simulink model "gm_slrt_pmsm_npc_inverter_slrt"  (R2022b)
settings: Solver=FixedStepAuto  StartTime=0.0  StopTime=0.25  RelTol=1e-3  EnableMultiTasking=on
PreLoadFcn:
  | Tcpu = 50e-6; %Controller sample time
  | 
  | % PMSM parameters
  | PM = 0.03; % Permanent magnet flux linkage
  | Ld = 2e-4;  % d-axis inductance
  | Lq = 2e-4;  % q-axis inductance
  | L0 = 2e-4;  % 0-axis inductance
  | Rs = 0.013; % Stator resistance
  | N = 6; % Number of pole pairs
  | J = 0.2; % Moment of inertia
  | 
  | % encoder parameters
  | numSlits = 2000; % number of slits
  | pulseSigOffset = 0; % index pulse signal offset
  | shaftInitPos = 0; % motor shaft initial position
  | 
  | % DAC parameters
  | gain = 0.1;
  | bias = 0;
  | 
  | % circuit parameters
  | Vdc = 48;
  | 
  | % Real-time processor or embedded controller
  | RTorTTL = 1; % 1: Real-time processor,    0: embedded controller
  | 
  | % real-time parameters
  | f_base = 200e6;
  | PWM_frequency = 20e3;
  | ts_FPGA_clk = 1/f_base;%5e-9
  | ts_FPGA_mdl =1e-6;
undefined symbols (not defined in the file or in its folder): IO334
libraries: speedgoatlib_hdlCoder_IO3xx x28, slrtencoderlib x1, slrtresolverlib x1
settings Model: Creator=chrisz  LastModifiedBy=chrisz
settings SolverCC: ConcurrentTasks=on  PositivePriorityOrder=on
settings OptimizationCC: BlockReduction=off  ConditionallyExecuteInputs=off  DefaultParameterBehavior=Inlined  OptimizeBlockIOStorage=off
settings DebuggingCC: AlgebraicLoopMsg=error  SingleTaskRateTransMsg=error  TasksWithSamePriorityMsg=none
settings HardwareCC: ProdBitPerLong=64  ProdLongLongMode=on  ProdHWDeviceType=Intel->x86-64 (Linux 64)  TargetBitPerPointer=64  TargetBitPerSizeT=64  TargetBitPerPtrDiffT=64  TargetLongLongMode=on  TargetIntDivRoundTo=Zero  TargetEndianess=LittleEndian  TargetWordSize=64  TargetHWDeviceType=Custom Processor->MATLAB Host Computer
settings ModelReferenceCC: EnableRefExpFcnMdlSchedulingChecks=on
settings RTWCC: Description=Simulink Real-Time  SystemTargetFile=slrealtime.tlc  TemplateMakefile=slrealtime_default_tmf  Toolchain=Simulink Real-Time Toolchain  BuildConfiguration=Faster Runs  CodeExecutionProfiling=on  TargetLang=C++

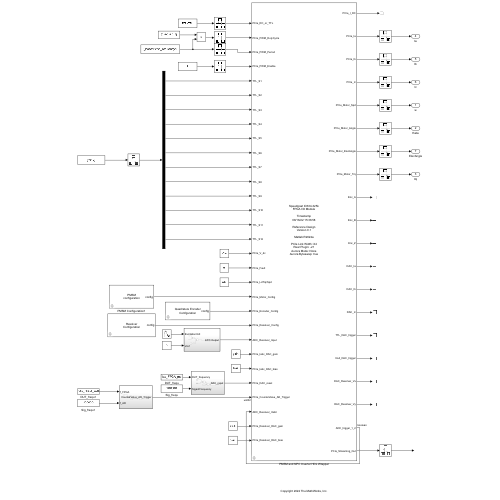
[thumbnail: Simulink's stored preview of the top-level diagram]
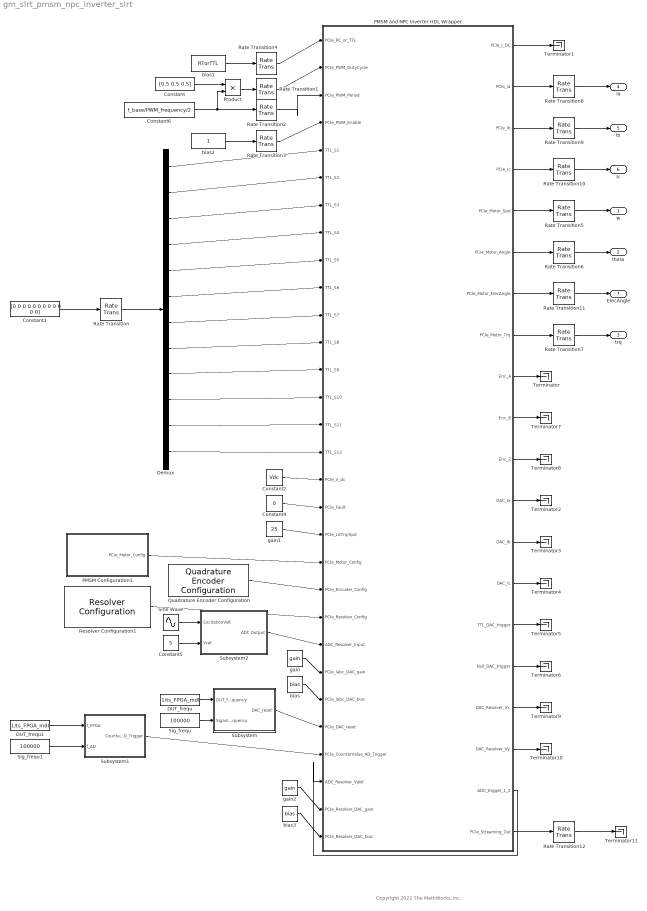
== system gm_slrt_pmsm_npc_inverter_slrt ==
  note: Copyright 2022 The MathWorks, Inc.
  Constant : Constant  Value=[0.5 0.5 0.5]  OutDataTypeStr=single  SampleTime=Tcpu
  Constant1 : Constant  Value=[0 0 0 0 0 0 0 0 0 0 0 0]  OutDataTypeStr=boolean  SampleTime=-1
  Constant2 : Constant  Value=Vdc  OutDataTypeStr=single  SampleTime=Tcpu
  Constant4 : Constant  Value=0  OutDataTypeStr=uint32  SampleTime=Tcpu
  Constant5 : Constant  Value=5  SampleTime=Tcpu
  Constant6 : Constant  Value=f_base/PWM_frequency/2  OutDataTypeStr=uint32  SampleTime=Tcpu
  DUT_frequ : Constant  Value=1/ts_FPGA_mdl  SampleTime=Tcpu
  DUT_frequ1 : Constant  Value=1/ts_FPGA_mdl  SampleTime=Tcpu
  Demux : Demux  Outputs=12
  PMSM Configuration1 : Subsystem  mask(PMSMConfig){portConfig=Torque, Trq_N_mode=0, Ts=Tcpu, Pp=4, Rs=0.02, Ld=1.7e-3, Lq=3.2e-3, lambda_pm=0.2205, J=0.0027, B=4.924e-4, f=0}
      mask prompts: portConfig "Mechanical input configuration:"; Ts "Sample time (s):"; Pp "Number of pole pairs:"; Rs "Stator resistance per phase (Ohm):"; Ld "Stator d-axis inductance (H):"; Lq "Stator q-axis inductance (H):"; lambda_pm "Permanent magnet flux linkage (Wb):"; J "Inertia (kgm^2):"; B "Viscous damping (Nm/rad/s):"; f "Static friction (Nm):"
      mask help: PMSM system configuration block
      mask TypeOptions portConfig: Torque | Speed
      mask Callback portConfig:
      | % Check the value selected in the pop-up
      | mask = Simulink.Mask.get(gcb);
      | portConfigStr = get_param(gcb, 'portConfig');
      | if strcmp(portConfigStr, 'Torque')
      |     % Set Trq_N_mode value to 0
      |     mask.getParameter('Trq_N_mode').Value = '0';
      | 
      | elseif strcmp(portConfigStr, 'Speed')
      |     % Set Trq_N_mode value to 2
      |     mask.getParameter('Trq_N_mode').Value = '1';
      | 
      | end
      mask DialogControl ParameterGroupVar Prompt: Block options
      mask DialogControl Container4 Prompt: Parameters
      mask Display:
      | disp('PMSM\nconfiguration');
      | port_label('output',1,'config');
  PMSM and NPC Inverter HDL Wrapper : Subsystem  mask(Speedgoat IO334-325k Interface Block){module_id=1, slot=-1, ts=-1, OutputRange=Auto (same as ADC), PullRPort0=pull-down, VioPort0=3.3V, PullRPort1=pull-down, VioPort1=3.3V, PullRPort2=pull-down, VioPort2=3.3V, PullRPort3=pull-down, VioPort3=3.3V, PullRPort4=pull-down, VioPort4=3.3V, PullRPort5=pull-down, VioPort5=3.3V, PullRPort6=pull-down, VioPort6=3.3V, FpgaFreq=200}
      mask prompts: module_id "FPGA Module Identifier:"; slot "PCI slot (-1: autosearch):"; ts "Sample time:"; OutputRange "DAC Voltage Range:"; PullRPort0 "pull resistor"; VioPort0 "I/O voltage"; PullRPort1 "pull resistor"; VioPort1 "I/O voltage"; PullRPort2 "pull resistor"; VioPort2 "I/O voltage"; PullRPort3 "pull resistor"; VioPort3 "I/O voltage"; PullRPort4 "pull resistor"; VioPort4 "I/O voltage"; PullRPort5 "pull resistor"; VioPort5 "I/O voltage"; PullRPort6 "pull resistor"; VioPort6 "I/O voltage"; FpgaFreq "FPGA Frequency [MHz]"
      mask help: Simulink Real-Time Interface Block for Speedgoat IO334-325k.
      mask init:
      | hdlslrt.backend.mfpgaparameters;
      mask Help: eval('speedgoatdoc_hdlc')
      mask TypeOptions OutputRange: IO334 DAC Setup/OutputRange
      mask TypeOptions PullRPort0: Port Settings -2x/PullRPort0
      mask Callback PullRPort0: sg_fpga_HDLCoder_io3xx_2x_m(2)
      mask TypeOptions VioPort0: Port Settings -2x/VioPort0
      mask Callback VioPort0: sg_fpga_HDLCoder_io3xx_2x_m(2)
      mask TypeOptions PullRPort1: Port Settings -2x/PullRPort1
      mask Callback PullRPort1: sg_fpga_HDLCoder_io3xx_2x_m(2)
      mask TypeOptions VioPort1: Port Settings -2x/VioPort1
      mask Callback VioPort1: sg_fpga_HDLCoder_io3xx_2x_m(2)
      mask TypeOptions PullRPort2: Port Settings -2x/PullRPort2
      mask Callback PullRPort2: sg_fpga_HDLCoder_io3xx_2x_m(2)
      mask TypeOptions VioPort2: Port Settings -2x/VioPort2
      mask Callback VioPort2: sg_fpga_HDLCoder_io3xx_2x_m(2)
      mask TypeOptions PullRPort3: Port Settings -2x/PullRPort3
      mask Callback PullRPort3: sg_fpga_HDLCoder_io3xx_2x_m(2)
      mask TypeOptions VioPort3: Port Settings -2x/VioPort3
      mask Callback VioPort3: sg_fpga_HDLCoder_io3xx_2x_m(2)
      mask TypeOptions PullRPort4: Port Settings -2x/PullRPort4
      mask Callback PullRPort4: sg_fpga_HDLCoder_io3xx_2x_m(2)
      mask TypeOptions VioPort4: Port Settings -2x/VioPort4
      mask Callback VioPort4: sg_fpga_HDLCoder_io3xx_2x_m(2)
      mask TypeOptions PullRPort5: Port Settings -2x/PullRPort5
      mask Callback PullRPort5: sg_fpga_HDLCoder_io3xx_2x_m(2)
      mask TypeOptions VioPort5: Port Settings -2x/VioPort5
      mask Callback VioPort5: sg_fpga_HDLCoder_io3xx_2x_m(2)
      mask TypeOptions PullRPort6: Port Settings -2x/PullRPort6
      mask Callback PullRPort6: sg_fpga_HDLCoder_io3xx_2x_m(2)
      mask TypeOptions VioPort6: Port Settings -2x/VioPort6
      mask Callback VioPort6: sg_fpga_HDLCoder_io3xx_2x_m(2)
      mask DialogControl AnalogOutput Prompt: Analog Output
      mask DialogControl IO33421 Prompt: IO334-21
      mask DialogControl port1 Prompt: Port 1
      mask DialogControl port2 Prompt: Port 2
      mask DialogControl port3 Prompt: Port 3
      mask DialogControl port4 Prompt: Port 4
      mask DialogControl port5 Prompt: Port 5
      mask DialogControl port6 Prompt: Port 6
      mask DialogControl port7 Prompt: Port 7
      mask Display:
      | SetupBlkPath = find_system(gcb, 'LookUnderMasks', 'all', 'FollowLinks', 'on', 'regexp', 'on', 'Name', 'IO3(\d|x){2}\s+Setup' );
      | SetupBlkPath = SetupBlkPath{1};
      | TS = get_param(SetupBlkPath,'timestamp_mcs');
      | disp(sprintf('Speedgoat IO334-325k\nFPGA I/O Module\n\nTimestamp\n%s\n\nReference Design\nVersion 0.1\n\nMatlab R2022a\n\nPCIe Link Width: X4\nRear Plugin: -21\nAurora Mode: None\nAurora Byteswap: true\n', TS))
  Product : Product  OutDataTypeStr=uint32
  Quadrature Encoder Configuration : slrtencoderlib/Quadrature Encoder Configuration  NPulses=2000  zOffset=0  Ts=Tcpu
  Rate Transition{,1..12} (13 alike) : RateTransition  OutPortSampleTime=Tcpu
  Resolver Configuration1 : slrtresolverlib/Resolver Configuration  Ts=Tcpu  R=0.5  N=1  ADCrefV=5  ADCbits=12  totalADCCounts=4096
  Sig_frequ : Constant  Value=100000  VectorParams1D=off  SampleTime=Tcpu
  Sig_frequ1 : Constant  Value=100000  VectorParams1D=off  SampleTime=Tcpu
  Sine Wave : Sin  Amplitude=5  Frequency=62830  SampleTime=Tcpu
  Subsystem : Subsystem
  Subsystem1 : Subsystem
  Subsystem2 : Subsystem
  Terminator{,1..11} (12 alike) : Terminator
  bias : Constant  Value=bias  OutDataTypeStr=single  SampleTime=Tcpu
  bias1 : Constant  Value=RTorTTL  OutDataTypeStr=single  SampleTime=Tcpu
  bias2 : Constant  OutDataTypeStr=boolean  SampleTime=Tcpu
  bias3 : Constant  Value=bias  OutDataTypeStr=single  SampleTime=Tcpu
  gain : Constant  Value=gain  OutDataTypeStr=single  SampleTime=Tcpu
  gain1 : Constant  Value=25  OutDataTypeStr=single  SampleTime=Tcpu
  gain2 : Constant  Value=gain  OutDataTypeStr=single  SampleTime=Tcpu
  w : Outport
  theta : Outport  Port=2
  trq : Outport  Port=3
  Ia : Outport  Port=4
  Ib : Outport  Port=5
  Ic : Outport  Port=6
  ElecAngle : Outport  Port=7
  wires:
  Rate Transition12/1 -> Terminator11/1
  PMSM and NPC Inverter HDL Wrapper/20(PCIe_Streaming_Out) -> Rate Transition12/1
  Rate Transition4/1 -> PMSM and NPC Inverter HDL Wrapper/1(PCIe_RC_or_TTL)
  Rate Transition1/1 -> PMSM and NPC Inverter HDL Wrapper/2(PCIe_PWM_DutyCycle)
  Rate Transition2/1 -> PMSM and NPC Inverter HDL Wrapper/3(PCIe_PWM_Period)
  Rate Transition3/1 -> PMSM and NPC Inverter HDL Wrapper/4(PCIe_PWM_Enable)
  Product/1 -> Rate Transition1/1
  Constant/1 -> Product/1
  bias2/1 -> Rate Transition3/1
  bias1/1 -> Rate Transition4/1
  Constant6/1 -> Rate Transition2/1, Product/2
  Demux/12 -> PMSM and NPC Inverter HDL Wrapper/16(TTL_S12)
  Demux/11 -> PMSM and NPC Inverter HDL Wrapper/15(TTL_S11)
  Demux/10 -> PMSM and NPC Inverter HDL Wrapper/14(TTL_S10)
  Demux/9 -> PMSM and NPC Inverter HDL Wrapper/13(TTL_S9)
  Demux/8 -> PMSM and NPC Inverter HDL Wrapper/12(TTL_S8)
  Demux/7 -> PMSM and NPC Inverter HDL Wrapper/11(TTL_S7)
  bias3/1 -> PMSM and NPC Inverter HDL Wrapper/30(PCIe_Resolver_DAC_bias)
  gain2/1 -> PMSM and NPC Inverter HDL Wrapper/29(PCIe_Resolver_DAC_gain)
  PMSM and NPC Inverter HDL Wrapper/7(PCIe_Motor_ElecAngle) -> Rate Transition11/1
  Rate Transition11/1 -> ElecAngle/1
  Subsystem2/1(ADC Output) -> PMSM and NPC Inverter HDL Wrapper/23(ADC_Resolver_Input)
  Constant5/1 -> Subsystem2/2(Vref)
  Sine Wave/1 -> Subsystem2/1(ExcitationVolt)
  DUT_frequ1/1 -> Subsystem1/1(f_FPGA)
  Sig_frequ1/1 -> Subsystem1/2(f_AD)
  PMSM and NPC Inverter HDL Wrapper/19(ADC_trigger_1_2) -> PMSM and NPC Inverter HDL Wrapper/28(ADC_Resolver_Valid)
  Subsystem1/1(CounterValue_AD_Trigger) -> PMSM and NPC Inverter HDL Wrapper/27(PCIe_CounterValue_AD_Trigger)
  Resolver Configuration1/1 -> PMSM and NPC Inverter HDL Wrapper/22(PCIe_Resolver_Config)
  PMSM Configuration1/1(PCIe_Motor_Config) -> PMSM and NPC Inverter HDL Wrapper/20(PCIe_Motor_Config)
  Quadrature Encoder Configuration/1 -> PMSM and NPC Inverter HDL Wrapper/21(PCIe_Encoder_Config)
  PMSM and NPC Inverter HDL Wrapper/18(DAC_Resolver_Vy) -> Terminator10/1
  PMSM and NPC Inverter HDL Wrapper/17(DAC_Resolver_Vx) -> Terminator9/1
  PMSM and NPC Inverter HDL Wrapper/11(Enc_Z) -> Terminator8/1
  PMSM and NPC Inverter HDL Wrapper/4(PCIe_Ic) -> Rate Transition10/1
  PMSM and NPC Inverter HDL Wrapper/3(PCIe_Ib) -> Rate Transition9/1
  PMSM and NPC Inverter HDL Wrapper/2(PCIe_Ia) -> Rate Transition8/1
  PMSM and NPC Inverter HDL Wrapper/8(PCIe_Motor_Trq) -> Rate Transition7/1
  PMSM and NPC Inverter HDL Wrapper/6(PCIe_Motor_Angle) -> Rate Transition6/1
  PMSM and NPC Inverter HDL Wrapper/5(PCIe_Motor_Spd) -> Rate Transition5/1
  Rate Transition8/1 -> Ia/1
  Rate Transition9/1 -> Ib/1
  PMSM and NPC Inverter HDL Wrapper/16(Null_DAC_trigger) -> Terminator6/1
  PMSM and NPC Inverter HDL Wrapper/13(DAC_Ib) -> Terminator3/1
  PMSM and NPC Inverter HDL Wrapper/15(TTL_DAC_trigger) -> Terminator5/1
  Rate Transition10/1 -> Ic/1
  Rate Transition5/1 -> w/1
  PMSM and NPC Inverter HDL Wrapper/14(DAC_Ic) -> Terminator4/1
  PMSM and NPC Inverter HDL Wrapper/10(Enc_B) -> Terminator7/1
  PMSM and NPC Inverter HDL Wrapper/1(PCIe_I_DC) -> Terminator1/1
  PMSM and NPC Inverter HDL Wrapper/12(DAC_Ia) -> Terminator2/1
  Rate Transition7/1 -> trq/1
  PMSM and NPC Inverter HDL Wrapper/9(Enc_A) -> Terminator/1
  Rate Transition6/1 -> theta/1
  Subsystem/1(DAC_reset) -> PMSM and NPC Inverter HDL Wrapper/26(PCIe_DAC_reset)
  Sig_frequ/1 -> Subsystem/2(SiganlFrequency)
  DUT_frequ/1 -> Subsystem/1(DUT_frequency)
  gain1/1 -> PMSM and NPC Inverter HDL Wrapper/19(PCIe_LdTrq/Spd)
  Constant4/1 -> PMSM and NPC Inverter HDL Wrapper/18(PCIe_Fault)
  Constant2/1 -> PMSM and NPC Inverter HDL Wrapper/17(PCIe_V_dc)
  Constant1/1 -> Rate Transition/1
  Demux/6 -> PMSM and NPC Inverter HDL Wrapper/10(TTL_S6)
  Demux/5 -> PMSM and NPC Inverter HDL Wrapper/9(TTL_S5)
  Demux/4 -> PMSM and NPC Inverter HDL Wrapper/8(TTL_S4)
  Demux/3 -> PMSM and NPC Inverter HDL Wrapper/7(TTL_S3)
  Demux/2 -> PMSM and NPC Inverter HDL Wrapper/6(TTL_S2)
  Demux/1 -> PMSM and NPC Inverter HDL Wrapper/5(TTL_S1)
  Rate Transition/1 -> Demux/1
  bias/1 -> PMSM and NPC Inverter HDL Wrapper/25(PCIe_Iabc_DAC_bias)
  gain/1 -> PMSM and NPC Inverter HDL Wrapper/24(PCIe_Iabc_DAC_gain)

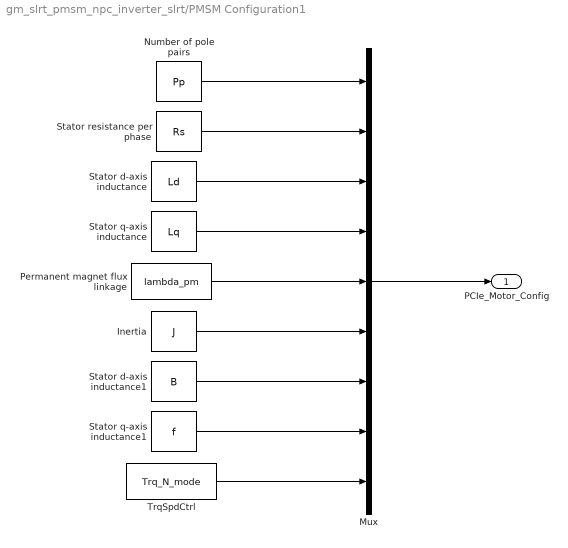
== system gm_slrt_pmsm_npc_inverter_slrt/PMSM Configuration1 ==
  Inertia : Constant  Value=J  OutDataTypeStr=single  SampleTime=Ts
  Mux : Mux  Inputs=9
  Number of pole pairs : Constant  Value=Pp  OutDataTypeStr=single  SampleTime=Ts
  Permanent magnet flux linkage : Constant  Value=lambda_pm  OutDataTypeStr=single  SampleTime=Ts
  Stator d-axis inductance : Constant  Value=Ld  OutDataTypeStr=single  SampleTime=Ts
  Stator d-axis inductance1 : Constant  Value=B  OutDataTypeStr=single  SampleTime=Ts
  Stator q-axis inductance : Constant  Value=Lq  OutDataTypeStr=single  SampleTime=Ts
  Stator q-axis inductance1 : Constant  Value=f  OutDataTypeStr=single  SampleTime=Ts
  Stator resistance per phase : Constant  Value=Rs  OutDataTypeStr=single  SampleTime=Ts
  TrqSpdCtrl : Constant  Value=Trq_N_mode  OutDataTypeStr=single  SampleTime=Ts
  PCIe_Motor_Config : Outport
  wires:
  Number of pole pairs/1 -> Mux/1
  Stator d-axis inductance/1 -> Mux/3
  Stator q-axis inductance/1 -> Mux/4
  Inertia/1 -> Mux/6
  Mux/1 -> PCIe_Motor_Config/1
  Stator d-axis inductance1/1 -> Mux/7
  Stator q-axis inductance1/1 -> Mux/8
  TrqSpdCtrl/1 -> Mux/9
  Stator resistance per phase/1 -> Mux/2
  Permanent magnet flux linkage/1 -> Mux/5

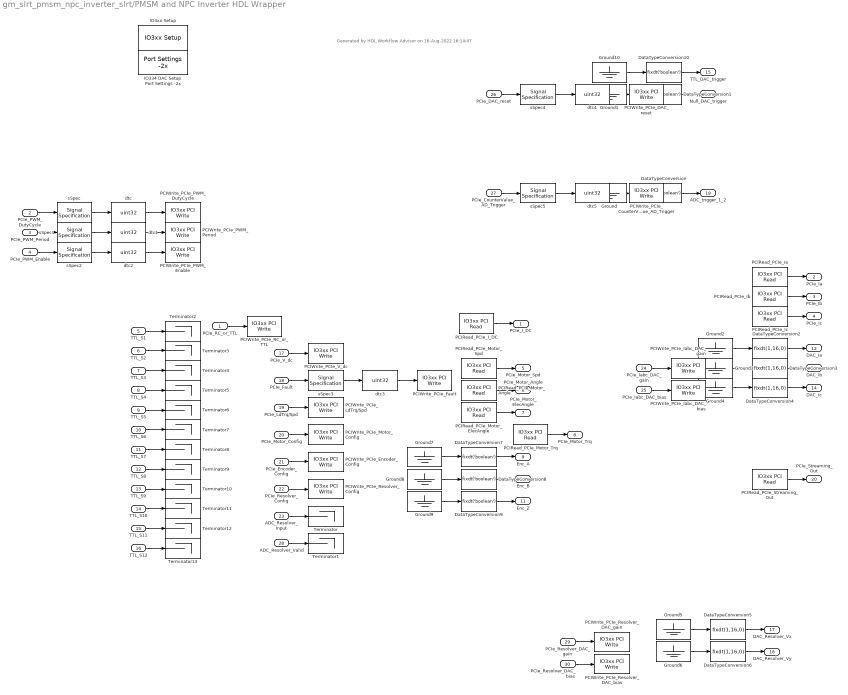
== system gm_slrt_pmsm_npc_inverter_slrt/PMSM and NPC Inverter HDL Wrapper ==
  note: Generated by HDL Workflow Advisor on 16-Aug-2022 16:14:47
  PCIe_RC_or_TTL : Inport
  PCIe_PWM_DutyCycle : Inport  Port=2
  PCIe_PWM_Period : Inport  Port=3
  PCIe_PWM_Enable : Inport  Port=4
  TTL_S1 : Inport  Port=5
  TTL_S2 : Inport  Port=6
  TTL_S3 : Inport  Port=7
  TTL_S4 : Inport  Port=8
  TTL_S5 : Inport  Port=9
  TTL_S6 : Inport  Port=10
  TTL_S7 : Inport  Port=11
  TTL_S8 : Inport  Port=12
  TTL_S9 : Inport  Port=13
  TTL_S10 : Inport  Port=14
  TTL_S11 : Inport  Port=15
  TTL_S12 : Inport  Port=16
  PCIe_V_dc : Inport  Port=17
  PCIe_Fault : Inport  Port=18
  PCIe_LdTrq/Spd : Inport  Port=19
  PCIe_Motor_Config : Inport  Port=20
  PCIe_Encoder_Config : Inport  Port=21
  PCIe_Resolver_Config : Inport  Port=22
  ADC_Resolver_Input : Inport  Port=23
  PCIe_Iabc_DAC_gain : Inport  Port=24
  PCIe_Iabc_DAC_bias : Inport  Port=25
  PCIe_DAC_reset : Inport  Port=26
  PCIe_CounterValue_AD_Trigger : Inport  Port=27  OutDataTypeStr=uint32
  ADC_Resolver_Valid : Inport  Port=28
  PCIe_Resolver_DAC_gain : Inport  Port=29
  PCIe_Resolver_DAC_bias : Inport  Port=30
  DataTypeConversion{,1,7..10} (6 alike) : DataTypeConversion  OutDataTypeStr=fixdt('boolean')  ConvertRealWorld=Stored Integer (SI)  SaturateOnIntegerOverflow=off  RndMeth=Floor
  DataTypeConversion{2..6} (5 alike) : DataTypeConversion  OutDataTypeStr=fixdt(1,16,0)  ConvertRealWorld=Stored Integer (SI)  SaturateOnIntegerOverflow=off  RndMeth=Floor
  Ground{,1..10} (11 alike) : Ground
  IO334 DAC Setup : speedgoatlib_hdlCoder_IO3xx/IO334 DAC Setup  module_id=module_id  OutputRange=Auto (same as ADC)
  IO3xx Setup : speedgoatlib_hdlCoder_IO3xx/IO3xx Setup  mdl_ss_name=slrt_pmsm_npc_inverter/PMSM and NPC Inverter HDL Wrapper  board_type=IO334-325k  fpga_sync_mode=on  reset_mode=on  reset_mode_stop=off  device_id=1  module_id=module_id  pci_slot=slot  fpga_mat_file=hdl_prj\hdlsrc\slrt_pmsm_npc_inverter\PMSMAndNPCInverterHDLWrapper.mat  timestamp_mcs=08/16/22 15:36:58  timestamp=2208161406  tsreg=hex2dec('8')  bsf_file=PMSMAndNPCInverterHDLWrapper.mcs  mcs=0
  PCIRead_PCIe_I_DC : speedgoatlib_hdlCoder_IO3xx/IO3xx PCI Read  device_id=1  module_id=module_id  board_type=IO334-325k  port_name=PCIe_I_DC  port_offset=hex2dec('1F0')  port_type=single  port_dim=3  strobe=hex2dec('200')  sample_time=ts
  PCIRead_PCIe_Ia : speedgoatlib_hdlCoder_IO3xx/IO3xx PCI Read  device_id=1  module_id=module_id  board_type=IO334-325k  port_name=PCIe_Ia  port_offset=hex2dec('18C')  port_type=single  port_dim=1  strobe=0  sample_time=ts
  PCIRead_PCIe_Ib : speedgoatlib_hdlCoder_IO3xx/IO3xx PCI Read  device_id=1  module_id=module_id  board_type=IO334-325k  port_name=PCIe_Ib  port_offset=hex2dec('1A4')  port_type=single  port_dim=1  strobe=0  sample_time=ts
  PCIRead_PCIe_Ic : speedgoatlib_hdlCoder_IO3xx/IO3xx PCI Read  device_id=1  module_id=module_id  board_type=IO334-325k  port_name=PCIe_Ic  port_offset=hex2dec('1A8')  port_type=single  port_dim=1  strobe=0  sample_time=ts
  PCIRead_PCIe_Motor_Angle : speedgoatlib_hdlCoder_IO3xx/IO3xx PCI Read  device_id=1  module_id=module_id  board_type=IO334-325k  port_name=PCIe_Motor_Angle  port_offset=hex2dec('1B0')  port_type=single  port_dim=1  strobe=0  sample_time=ts
  PCIRead_PCIe_Motor_ElecAngle : speedgoatlib_hdlCoder_IO3xx/IO3xx PCI Read  device_id=1  module_id=module_id  board_type=IO334-325k  port_name=PCIe_Motor_ElecAngle  port_offset=hex2dec('1BC')  port_type=single  port_dim=1  strobe=0  sample_time=ts
  PCIRead_PCIe_Motor_Spd : speedgoatlib_hdlCoder_IO3xx/IO3xx PCI Read  device_id=1  module_id=module_id  board_type=IO334-325k  port_name=PCIe_Motor_Spd  port_offset=hex2dec('1AC')  port_type=single  port_dim=1  strobe=0  sample_time=ts
  PCIRead_PCIe_Motor_Trq : speedgoatlib_hdlCoder_IO3xx/IO3xx PCI Read  device_id=1  module_id=module_id  board_type=IO334-325k  port_name=PCIe_Motor_Trq  port_offset=hex2dec('10C')  port_type=single  port_dim=1  strobe=0  sample_time=ts
  PCIRead_PCIe_Streaming_Out : speedgoatlib_hdlCoder_IO3xx/IO3xx PCI Read  device_id=1  module_id=module_id  board_type=IO334-325k  port_name=PCIe_Streaming_Out  port_offset=hex2dec('800')  port_type=single  port_dim=150  strobe=hex2dec('C00')  sample_time=ts
  PCIWrite_PCIe_CounterValue_AD_Trigger : speedgoatlib_hdlCoder_IO3xx/IO3xx PCI Write  device_id=1  module_id=module_id  board_type=IO334-325k  port_name=PCIe_CounterValue_AD_Trigger  port_offset=hex2dec('184')  port_type=uint32  port_dim=1  strobe=0  sample_time=ts
  PCIWrite_PCIe_DAC_reset : speedgoatlib_hdlCoder_IO3xx/IO3xx PCI Write  device_id=1  module_id=module_id  board_type=IO334-325k  port_name=PCIe_DAC_reset  port_offset=hex2dec('13C')  port_type=uint32  port_dim=1  strobe=0  sample_time=ts
  PCIWrite_PCIe_Encoder_Config : speedgoatlib_hdlCoder_IO3xx/IO3xx PCI Write  device_id=1  module_id=module_id  board_type=IO334-325k  port_name=PCIe_Encoder_Config  port_offset=hex2dec('190')  port_type=single  port_dim=3  strobe=hex2dec('1A0')  sample_time=ts
  PCIWrite_PCIe_Fault : speedgoatlib_hdlCoder_IO3xx/IO3xx PCI Write  device_id=1  module_id=module_id  board_type=IO334-325k  port_name=PCIe_Fault  port_offset=hex2dec('12C')  port_type=uint32  port_dim=1  strobe=0  sample_time=ts
  PCIWrite_PCIe_Iabc_DAC_bias : speedgoatlib_hdlCoder_IO3xx/IO3xx PCI Write  device_id=1  module_id=module_id  board_type=IO334-325k  port_name=PCIe_Iabc_DAC_bias  port_offset=hex2dec('138')  port_type=single  port_dim=1  strobe=0  sample_time=ts
  PCIWrite_PCIe_Iabc_DAC_gain : speedgoatlib_hdlCoder_IO3xx/IO3xx PCI Write  device_id=1  module_id=module_id  board_type=IO334-325k  port_name=PCIe_Iabc_DAC_gain  port_offset=hex2dec('134')  port_type=single  port_dim=1  strobe=0  sample_time=ts
  PCIWrite_PCIe_LdTrq/Spd : speedgoatlib_hdlCoder_IO3xx/IO3xx PCI Write  device_id=1  module_id=module_id  board_type=IO334-325k  port_name=PCIe_LdTrq//Spd  port_offset=hex2dec('130')  port_type=single  port_dim=1  strobe=0  sample_time=ts
  PCIWrite_PCIe_Motor_Config : speedgoatlib_hdlCoder_IO3xx/IO3xx PCI Write  device_id=1  module_id=module_id  board_type=IO334-325k  port_name=PCIe_Motor_Config  port_offset=hex2dec('140')  port_type=single  port_dim=9  strobe=hex2dec('180')  sample_time=ts
  PCIWrite_PCIe_PWM_DutyCycle : speedgoatlib_hdlCoder_IO3xx/IO3xx PCI Write  device_id=1  module_id=module_id  board_type=IO334-325k  port_name=PCIe_PWM_DutyCycle  port_offset=hex2dec('110')  port_type=uint32  port_dim=3  strobe=hex2dec('120')  sample_time=ts
  PCIWrite_PCIe_PWM_Enable : speedgoatlib_hdlCoder_IO3xx/IO3xx PCI Write  device_id=1  module_id=module_id  board_type=IO334-325k  port_name=PCIe_PWM_Enable  port_offset=hex2dec('108')  port_type=uint32  port_dim=1  strobe=0  sample_time=ts
  PCIWrite_PCIe_PWM_Period : speedgoatlib_hdlCoder_IO3xx/IO3xx PCI Write  device_id=1  module_id=module_id  board_type=IO334-325k  port_name=PCIe_PWM_Period  port_offset=hex2dec('104')  port_type=uint32  port_dim=1  strobe=0  sample_time=ts
  PCIWrite_PCIe_RC_or_TTL : speedgoatlib_hdlCoder_IO3xx/IO3xx PCI Write  device_id=1  module_id=module_id  board_type=IO334-325k  port_name=PCIe_RC_or_TTL  port_offset=hex2dec('100')  port_type=single  port_dim=1  strobe=0  sample_time=ts
  PCIWrite_PCIe_Resolver_Config : speedgoatlib_hdlCoder_IO3xx/IO3xx PCI Write  device_id=1  module_id=module_id  board_type=IO334-325k  port_name=PCIe_Resolver_Config  port_offset=hex2dec('1C0')  port_type=single  port_dim=6  strobe=hex2dec('1E0')  sample_time=ts
  PCIWrite_PCIe_Resolver_DAC_bias : speedgoatlib_hdlCoder_IO3xx/IO3xx PCI Write  device_id=1  module_id=module_id  board_type=IO334-325k  port_name=PCIe_Resolver_DAC_bias  port_offset=hex2dec('1B8')  port_type=single  port_dim=1  strobe=0  sample_time=ts
  PCIWrite_PCIe_Resolver_DAC_gain : speedgoatlib_hdlCoder_IO3xx/IO3xx PCI Write  device_id=1  module_id=module_id  board_type=IO334-325k  port_name=PCIe_Resolver_DAC_gain  port_offset=hex2dec('1B4')  port_type=single  port_dim=1  strobe=0  sample_time=ts
  PCIWrite_PCIe_V_dc : speedgoatlib_hdlCoder_IO3xx/IO3xx PCI Write  device_id=1  module_id=module_id  board_type=IO334-325k  port_name=PCIe_V_dc  port_offset=hex2dec('128')  port_type=single  port_dim=1  strobe=0  sample_time=ts
  Port Settings -2x : speedgoatlib_hdlCoder_IO3xx/Port Settings -2x  module_id=module_id  rearIO=-21  PullRPort0=pull-down  VioPort0=3.3V  PullRPort1=pull-down  VioPort1=3.3V  PullRPort2=pull-down  VioPort2=3.3V  PullRPort3=pull-down  VioPort3=3.3V  PullRPort4=pull-down  VioPort4=3.3V  PullRPort5=pull-down  VioPort5=3.3V  PullRPort6=pull-down  VioPort6=3.3V
  Terminator{,1..13} (14 alike) : Terminator
  dtc{,1..5} (6 alike) : DataTypeConversion  OutDataTypeStr=uint32  ConvertRealWorld=Stored Integer (SI)  SaturateOnIntegerOverflow=off
  sSpec{,1,3,5} (4 alike) : SignalSpecification  OutDataTypeStr=fixdt(0,32,0)
  sSpec2 : SignalSpecification  OutDataTypeStr=fixdt('boolean')
  sSpec4 : SignalSpecification  OutDataTypeStr=fixdt(0,16,0)
  PCIe_I_DC : Outport
  PCIe_Ia : Outport  Port=2
  PCIe_Ib : Outport  Port=3
  PCIe_Ic : Outport  Port=4
  PCIe_Motor_Spd : Outport  Port=5
  PCIe_Motor_Angle : Outport  Port=6
  PCIe_Motor_ElecAngle : Outport  Port=7
  PCIe_Motor_Trq : Outport  Port=8
  Enc_A : Outport  Port=9
  Enc_B : Outport  Port=10
  Enc_Z : Outport  Port=11
  DAC_Ia : Outport  Port=12
  DAC_Ib : Outport  Port=13
  DAC_Ic : Outport  Port=14
  TTL_DAC_trigger : Outport  Port=15
  Null_DAC_trigger : Outport  Port=16
  DAC_Resolver_Vx : Outport  Port=17
  DAC_Resolver_Vy : Outport  Port=18
  ADC_trigger_1_2 : Outport  Port=19  OutDataTypeStr=boolean
  PCIe_Streaming_Out : Outport  Port=20
  wires:
  PCIe_RC_or_TTL/1 -> PCIWrite_PCIe_RC_or_TTL/1
  PCIe_PWM_DutyCycle/1 -> sSpec/1
  sSpec/1 -> dtc/1
  dtc/1 -> PCIWrite_PCIe_PWM_DutyCycle/1
  PCIe_PWM_Period/1 -> sSpec1/1
  sSpec1/1 -> dtc1/1
  dtc1/1 -> PCIWrite_PCIe_PWM_Period/1
  PCIe_PWM_Enable/1 -> sSpec2/1
  sSpec2/1 -> dtc2/1
  dtc2/1 -> PCIWrite_PCIe_PWM_Enable/1
  PCIe_V_dc/1 -> PCIWrite_PCIe_V_dc/1
  PCIe_Fault/1 -> sSpec3/1
  sSpec3/1 -> dtc3/1
  dtc3/1 -> PCIWrite_PCIe_Fault/1
  PCIe_LdTrq/Spd/1 -> PCIWrite_PCIe_LdTrq/Spd/1
  PCIe_Motor_Config/1 -> PCIWrite_PCIe_Motor_Config/1
  PCIe_Encoder_Config/1 -> PCIWrite_PCIe_Encoder_Config/1
  PCIe_Resolver_Config/1 -> PCIWrite_PCIe_Resolver_Config/1
  PCIe_Iabc_DAC_gain/1 -> PCIWrite_PCIe_Iabc_DAC_gain/1
  PCIe_Iabc_DAC_bias/1 -> PCIWrite_PCIe_Iabc_DAC_bias/1
  PCIe_DAC_reset/1 -> sSpec4/1
  sSpec4/1 -> dtc4/1
  dtc4/1 -> PCIWrite_PCIe_DAC_reset/1
  PCIe_CounterValue_AD_Trigger/1 -> sSpec5/1
  sSpec5/1 -> dtc5/1
  dtc5/1 -> PCIWrite_PCIe_CounterValue_AD_Trigger/1
  PCIe_Resolver_DAC_gain/1 -> PCIWrite_PCIe_Resolver_DAC_gain/1
  PCIe_Resolver_DAC_bias/1 -> PCIWrite_PCIe_Resolver_DAC_bias/1
  PCIRead_PCIe_I_DC/1 -> PCIe_I_DC/1
  PCIRead_PCIe_Ia/1 -> PCIe_Ia/1
  PCIRead_PCIe_Ib/1 -> PCIe_Ib/1
  PCIRead_PCIe_Ic/1 -> PCIe_Ic/1
  PCIRead_PCIe_Motor_Spd/1 -> PCIe_Motor_Spd/1
  PCIRead_PCIe_Motor_Angle/1 -> PCIe_Motor_Angle/1
  PCIRead_PCIe_Motor_ElecAngle/1 -> PCIe_Motor_ElecAngle/1
  PCIRead_PCIe_Motor_Trq/1 -> PCIe_Motor_Trq/1
  PCIRead_PCIe_Streaming_Out/1 -> PCIe_Streaming_Out/1
  ADC_Resolver_Input/1 -> Terminator/1
  ADC_Resolver_Valid/1 -> Terminator1/1
  DataTypeConversion/1 -> ADC_trigger_1_2/1
  Ground/1 -> DataTypeConversion/1
  DataTypeConversion1/1 -> Null_DAC_trigger/1
  Ground1/1 -> DataTypeConversion1/1
  DataTypeConversion2/1 -> DAC_Ia/1
  Ground2/1 -> DataTypeConversion2/1
  DataTypeConversion3/1 -> DAC_Ib/1
  Ground3/1 -> DataTypeConversion3/1
  DataTypeConversion4/1 -> DAC_Ic/1
  Ground4/1 -> DataTypeConversion4/1
  DataTypeConversion5/1 -> DAC_Resolver_Vx/1
  Ground5/1 -> DataTypeConversion5/1
  DataTypeConversion6/1 -> DAC_Resolver_Vy/1
  Ground6/1 -> DataTypeConversion6/1
  TTL_S1/1 -> Terminator2/1
  TTL_S2/1 -> Terminator3/1
  TTL_S3/1 -> Terminator4/1
  TTL_S4/1 -> Terminator5/1
  TTL_S5/1 -> Terminator6/1
  TTL_S6/1 -> Terminator7/1
  TTL_S7/1 -> Terminator8/1
  TTL_S8/1 -> Terminator9/1
  TTL_S9/1 -> Terminator10/1
  TTL_S10/1 -> Terminator11/1
  TTL_S11/1 -> Terminator12/1
  TTL_S12/1 -> Terminator13/1
  DataTypeConversion7/1 -> Enc_A/1
  Ground7/1 -> DataTypeConversion7/1
  DataTypeConversion8/1 -> Enc_B/1
  Ground8/1 -> DataTypeConversion8/1
  DataTypeConversion9/1 -> Enc_Z/1
  Ground9/1 -> DataTypeConversion9/1
  DataTypeConversion10/1 -> TTL_DAC_trigger/1
  Ground10/1 -> DataTypeConversion10/1

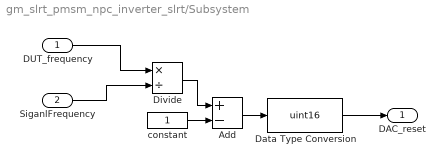
== system gm_slrt_pmsm_npc_inverter_slrt/Subsystem ==
  DUT_frequency : Inport
  SiganlFrequency : Inport  Port=2
  Add : Sum  Inputs=+-
  Data Type Conversion : DataTypeConversion  OutDataTypeStr=uint16  SaturateOnIntegerOverflow=off  RndMeth=Floor
  Divide : Product  Inputs=*/
  constant : Constant  VectorParams1D=off  SampleTime=-1
  DAC_reset : Outport
  wires:
  SiganlFrequency/1 -> Divide/2
  Add/1 -> Data Type Conversion/1
  Divide/1 -> Add/1
  Data Type Conversion/1 -> DAC_reset/1
  constant/1 -> Add/2
  DUT_frequency/1 -> Divide/1

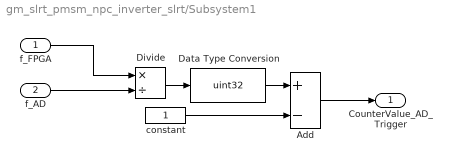
== system gm_slrt_pmsm_npc_inverter_slrt/Subsystem1 ==
  f_FPGA : Inport
  f_AD : Inport  Port=2
  Add : Sum  Inputs=+-  AccumDataTypeStr=uint32
  Data Type Conversion : DataTypeConversion  OutDataTypeStr=uint32  SaturateOnIntegerOverflow=off  RndMeth=Floor
  Divide : Product  Inputs=*/
  constant : Constant  VectorParams1D=off  OutDataTypeStr=uint32  SampleTime=-1
  CounterValue_AD_Trigger : Outport
  wires:
  Add/1 -> CounterValue_AD_Trigger/1
  constant/1 -> Add/2
  Data Type Conversion/1 -> Add/1
  Divide/1 -> Data Type Conversion/1
  f_FPGA/1 -> Divide/1
  f_AD/1 -> Divide/2

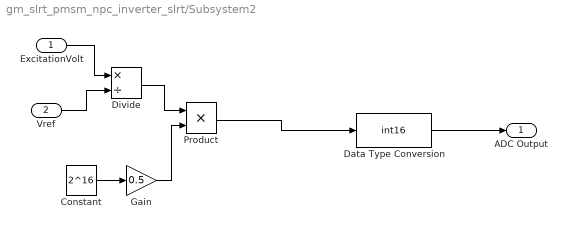
== system gm_slrt_pmsm_npc_inverter_slrt/Subsystem2 ==
  ExcitationVolt : Inport
  Vref : Inport  Port=2
  Constant : Constant  Value=2^16  SampleTime=-1
  Data Type Conversion : DataTypeConversion  OutDataTypeStr=int16  RndMeth=Nearest
  Divide : Product  Inputs=*/
  Gain : Gain  Gain=0.5
  Product : Product
  ADC Output : Outport
  wires:
  Data Type Conversion/1 -> ADC Output/1
  Product/1 -> Data Type Conversion/1
  Gain/1 -> Product/2
  Divide/1 -> Product/1
  Constant/1 -> Gain/1
  Vref/1 -> Divide/2
  ExcitationVolt/1 -> Divide/1
